simulink model "FW_Matlab_main"  (R2024b)
settings: Solver=ode4  StartTime=0.0  StopTime=inf  FixedStep=0.001  RelTol=1e-3
model workspace (MAT data in the model file):
  freq = 1
libraries: eeGeneralControl x8, slrealtimeiplib x5, cstblocks x3, simulink_extras x2, vrlib x1, aerolibanimutils x1, dspnetwork x1
(part 2 of 2)

== matlab function FW_Matlab_main/普通扑翼/MATLAB Function1 ==
  data: t input; y output
function y = back_flap(t)
%y=30+60*cos((226.08*t+180)*(pi/180));
y=60*cos((226.08*t+180)*(pi/180));
end

== matlab function FW_Matlab_main/普通扑翼/MATLAB Function2 ==
  data: t input; y output
function y = back_flap_twist(t)
  sita_u=90+30;   %上扑角度
  sita_d=90-30;   %下扑角度
  delta_T=0.4;
  T=1.6;
  sita_b_value=0;
  if t>=-delta_T/2 && t<=delta_T/2
    sita_b_value=(sita_u+sita_d)/2+((sita_u-sita_d)/2)*sin(3.14*t/delta_T);
  end
   if t>=delta_T/2 && t<=(T-delta_T)/2
    sita_b_value=sita_u;
   end
   if t>=(T-delta_T)/2 && t<=(T+delta_T)/2
    sita_b_value=(sita_u+sita_d)/2+((sita_u-sita_d)/2)*sin(3.14*(T/2-t)/delta_T);
   end
   if t>=(T+delta_T)/2 && t<=T-delta_T/2
    sita_b_value=sita_d;
   end
   if t>=T-delta_T/2 && t<=T
    sita_b_value=(sita_u+sita_d)/2+((sita_u-sita_d)/2)*sin(3.14*t/delta_T);
   end
   y=sita_b_value;
end

== matlab function FW_Matlab_main/普通扑翼/MATLAB Function3 ==
  data: t input; y output
function y = back_flap_twist(t)
  sita_u=90+30;   %上扑角度
  sita_d=90-30;   %下扑角度
  delta_T=0.4;
  T=1.6;
  sita_b_value=0;
  if t>=-delta_T/2 && t<=delta_T/2
    sita_b_value=(sita_u+sita_d)/2+((sita_u-sita_d)/2)*sin(3.14*t/delta_T);
  end
   if t>=delta_T/2 && t<=(T-delta_T)/2
    sita_b_value=sita_u;
   end
   if t>=(T-delta_T)/2 && t<=(T+delta_T)/2
    sita_b_value=(sita_u+sita_d)/2+((sita_u-sita_d)/2)*sin(3.14*(T/2-t)/delta_T);
   end
   if t>=(T+delta_T)/2 && t<=T-delta_T/2
    sita_b_value=sita_d;
   end
   if t>=T-delta_T/2 && t<=T
    sita_b_value=(sita_u+sita_d)/2+((sita_u-sita_d)/2)*sin(3.14*t/delta_T);
   end
   y=sita_b_value;
end

== matlab function FW_Matlab_main/Saw_Tooth ==
  data: freq input; Out output; t input
function Out = Saw_Tooth(freq,t)
% 设置参数
frequency = freq; % 频率
amplitude = 1 % 幅度

% 生成锯齿波形
Out = (sawtooth(2*pi*frequency*t, amplitude)+1)/2;

== matlab function FW_Matlab_main/蜻蜓扑动-VTOL模式 45度范围/MATLAB Function3 ==
  data: t input; y output
function y = back_flap_twist(t)
  sita_u=170;   %上扑角度
  sita_d=65;   %下扑角度
  delta_T=0.4;
  T=1.6;
  sita_b_value=0;
  if t>=-delta_T/2 && t<=delta_T/2
    sita_b_value=(sita_u+sita_d)/2+((sita_u-sita_d)/2)*sin(3.14*t/delta_T);
  end
   if t>=delta_T/2 && t<=(T-delta_T)/2
    sita_b_value=sita_u;
   end
   if t>=(T-delta_T)/2 && t<=(T+delta_T)/2
    sita_b_value=(sita_u+sita_d)/2+((sita_u-sita_d)/2)*sin(3.14*(T/2-t)/delta_T);
   end
   if t>=(T+delta_T)/2 && t<=T-delta_T/2
    sita_b_value=sita_d;
   end
   if t>=T-delta_T/2 && t<=T
    sita_b_value=(sita_u+sita_d)/2+((sita_u-sita_d)/2)*sin(3.14*t/delta_T);
   end
   y=sita_b_value;
end

== matlab function FW_Matlab_main/Saw_Tooth1 ==
  data: freq input; Out output; t input
function Out = Saw_Tooth(freq,t)
% 设置参数
frequency = freq; % 频率
amplitude = 1 % 幅度

% 生成锯齿波形
Out = (sawtooth(2*pi*frequency*t, amplitude)+1)/2;

== matlab function FW_Matlab_main/MATLAB Function ==
  data: Azimuth_Angle input; Freq_diff_out output; force_req_x input; force_req_y input
function Freq_diff_out = Flapping_Freq_Change(Azimuth_Angle,force_req_x,force_req_y)
%% 处理x轴
change_x=force_req_x/sind(Azimuth_Angle);
if isnan(change_x)
    change_x=0;
end
if isinf(change_x)
    change_x=0;
end

if abs(change_x)>10
  change_x=10;
end
Freq_diff_out_x=change_x;
%% 处理y轴
change_y=-force_req_y/cosd(Azimuth_Angle);
if isnan(change_y)
    change_y=0;
end
if isinf(change_y)
    change_y=0;
end

if abs(change_y)>10
  change_y=10;
end
Freq_diff_out_y=change_y;

Freq_diff_out=Freq_diff_out_x+Freq_diff_out_y;
if Freq_diff_out>=2.5
  Freq_diff_out=2.5;
end
if Freq_diff_out<=-2.5
  Freq_diff_out=-2.5;
end
end

== matlab function FW_Matlab_main/论文模式 FWR（拍幅：10//-10 扭转角5//25）Cl5.11? 升力没论文说的大 1/MATLAB Function ==
  data: t input; y output
function y = back_flap(t)
y=10*cos((226.08*t+180)*(pi/180));
end

== matlab function FW_Matlab_main/论文模式 FWR（拍幅：10//-10 扭转角5//25）Cl5.11? 升力没论文说的大 1/MATLAB Function1 ==
  data: t input; y output
function y = back_flap(t)
y=10*cos((226.08*t+180)*(pi/180));
end

== matlab function FW_Matlab_main/论文模式 FWR（拍幅：10//-10 扭转角5//25）Cl5.11? 升力没论文说的大 1/MATLAB Function2 ==
  data: t input; y output
function y = back_flap_twist(t)
  sita_u=90+25;   %上扑角度
  sita_d=90+5;   %下扑角度
  delta_T=0.4;
  T=1.6;
  sita_b_value=0;
  if t>=-delta_T/2 && t<=delta_T/2
    sita_b_value=(sita_u+sita_d)/2+((sita_u-sita_d)/2)*sin(3.14*t/delta_T);
  end
   if t>=delta_T/2 && t<=(T-delta_T)/2
    sita_b_value=sita_u;
   end
   if t>=(T-delta_T)/2 && t<=(T+delta_T)/2
    sita_b_value=(sita_u+sita_d)/2+((sita_u-sita_d)/2)*sin(3.14*(T/2-t)/delta_T);
   end
   if t>=(T+delta_T)/2 && t<=T-delta_T/2
    sita_b_value=sita_d;
   end
   if t>=T-delta_T/2 && t<=T
    sita_b_value=(sita_u+sita_d)/2+((sita_u-sita_d)/2)*sin(3.14*t/delta_T);
   end
   y=sita_b_value;
end

== matlab function FW_Matlab_main/论文模式 FWR（拍幅：10//-10 扭转角5//25）Cl5.11? 升力没论文说的大 1/MATLAB Function3 ==
  data: t input; y output
function y = back_flap_twist(t)
  sita_u=90+25;   %上扑角度
  sita_d=90+5;   %下扑角度
  delta_T=0.4;
  T=1.6;
  sita_b_value=0;
  if t>=-delta_T/2 && t<=delta_T/2
    sita_b_value=(sita_u+sita_d)/2+((sita_u-sita_d)/2)*sin(3.14*t/delta_T);
  end
   if t>=delta_T/2 && t<=(T-delta_T)/2
    sita_b_value=sita_u;
   end
   if t>=(T-delta_T)/2 && t<=(T+delta_T)/2
    sita_b_value=(sita_u+sita_d)/2+((sita_u-sita_d)/2)*sin(3.14*(T/2-t)/delta_T);
   end
   if t>=(T+delta_T)/2 && t<=T-delta_T/2
    sita_b_value=sita_d;
   end
   if t>=T-delta_T/2 && t<=T
    sita_b_value=(sita_u+sita_d)/2+((sita_u-sita_d)/2)*sin(3.14*t/delta_T);
   end
   y=sita_b_value;
end

== matlab function FW_Matlab_main/优化中 FWR（当前最优）10.29前/MATLAB Function ==
  data: t input; y output
function y = back_flap(t)
y=30+60*cos((226.08*t+180)*(pi/180));
end

== matlab function FW_Matlab_main/优化中 FWR（当前最优）10.29前/MATLAB Function1 ==
  data: t input; y output
function y = back_flap(t)
y=30+60*cos((226.08*t+180)*(pi/180));
end

== matlab function FW_Matlab_main/优化中 FWR（当前最优）10.29前/MATLAB Function2 ==
  data: t input; y output
function y = back_flap_twist(t)
  sita_u=90+45;   %上扑角度
  sita_d=90-5;   %下扑角度
  delta_T=0.4;
  T=1.6;
  sita_b_value=0;
  if t>=-delta_T/2 && t<=delta_T/2
    sita_b_value=(sita_u+sita_d)/2+((sita_u-sita_d)/2)*sin(3.14*t/delta_T);
  end
   if t>=delta_T/2 && t<=(T-delta_T)/2
    sita_b_value=sita_u;
   end
   if t>=(T-delta_T)/2 && t<=(T+delta_T)/2
    sita_b_value=(sita_u+sita_d)/2+((sita_u-sita_d)/2)*sin(3.14*(T/2-t)/delta_T);
   end
   if t>=(T+delta_T)/2 && t<=T-delta_T/2
    sita_b_value=sita_d;
   end
   if t>=T-delta_T/2 && t<=T
    sita_b_value=(sita_u+sita_d)/2+((sita_u-sita_d)/2)*sin(3.14*t/delta_T);
   end
   y=sita_b_value;
end

== matlab function FW_Matlab_main/蜻蜓扑动-FWR模式-角度与普通蜻蜓同  45度范围/MATLAB Function ==
  data: t input; y output
function y = back_flap(t)
y=15+30*cos((226.08*t+180)*(pi/180));
end

== matlab function FW_Matlab_main/优化中 FWR（当前最优）10.29前/MATLAB Function3 ==
  data: t input; y output
function y = back_flap_twist(t)
  sita_u=90+45;   %上扑角度
  sita_d=90-5;   %下扑角度
  delta_T=0.4;
  T=1.6;
  sita_b_value=0;
  if t>=-delta_T/2 && t<=delta_T/2
    sita_b_value=(sita_u+sita_d)/2+((sita_u-sita_d)/2)*sin(3.14*t/delta_T);
  end
   if t>=delta_T/2 && t<=(T-delta_T)/2
    sita_b_value=sita_u;
   end
   if t>=(T-delta_T)/2 && t<=(T+delta_T)/2
    sita_b_value=(sita_u+sita_d)/2+((sita_u-sita_d)/2)*sin(3.14*(T/2-t)/delta_T);
   end
   if t>=(T+delta_T)/2 && t<=T-delta_T/2
    sita_b_value=sita_d;
   end
   if t>=T-delta_T/2 && t<=T
    sita_b_value=(sita_u+sita_d)/2+((sita_u-sita_d)/2)*sin(3.14*t/delta_T);
   end
   y=sita_b_value;
end

== matlab function FW_Matlab_main/蜻蜓扑动-FWR模式-角度与普通蜻蜓同  45度范围/MATLAB Function1 ==
  data: t input; y output
function y = back_flap(t)
y=15+30*cos((226.08*t+180)*(pi/180));
end

== matlab function FW_Matlab_main/MATLAB Function6 ==
  data: Lift input; Cl output; freq input; Amp input
function Cl = Cl_cal(Lift,freq,Amp)
%初始参数设定
S=15*(1/100)*5.5*(1/100);
R2=0.5*18*(1/100);
Uref=2*deg2rad(Amp)*freq*R2;
air_p=1.225;
Cl=Lift*(1/1000)/(0.5*air_p*(Uref^2)*S);
end

== matlab function FW_Matlab_main/蜻蜓扑动-FWR模式-角度与普通蜻蜓同  45度范围/MATLAB Function2 ==
  data: t input; y output
function y = back_flap_twist(t)
  sita_u=170;   %上扑角度
  sita_d=65;   %下扑角度
  delta_T=0.4;
  T=1.6;
  sita_b_value=0;
  if t>=-delta_T/2 && t<=delta_T/2
    sita_b_value=(sita_u+sita_d)/2+((sita_u-sita_d)/2)*sin(3.14*t/delta_T);
  end
   if t>=delta_T/2 && t<=(T-delta_T)/2
    sita_b_value=sita_u;
   end
   if t>=(T-delta_T)/2 && t<=(T+delta_T)/2
    sita_b_value=(sita_u+sita_d)/2+((sita_u-sita_d)/2)*sin(3.14*(T/2-t)/delta_T);
   end
   if t>=(T+delta_T)/2 && t<=T-delta_T/2
    sita_b_value=sita_d;
   end
   if t>=T-delta_T/2 && t<=T
    sita_b_value=(sita_u+sita_d)/2+((sita_u-sita_d)/2)*sin(3.14*t/delta_T);
   end
   y=sita_b_value;
end

== matlab function FW_Matlab_main/蜻蜓扑动-FWR模式-角度与普通蜻蜓同  45度范围/MATLAB Function3 ==
  data: t input; y output
function y = back_flap_twist(t)
  sita_u=170;   %上扑角度
  sita_d=65;   %下扑角度
  delta_T=0.4;
  T=1.6;
  sita_b_value=0;
  if t>=-delta_T/2 && t<=delta_T/2
    sita_b_value=(sita_u+sita_d)/2+((sita_u-sita_d)/2)*sin(3.14*t/delta_T);
  end
   if t>=delta_T/2 && t<=(T-delta_T)/2
    sita_b_value=sita_u;
   end
   if t>=(T-delta_T)/2 && t<=(T+delta_T)/2
    sita_b_value=(sita_u+sita_d)/2+((sita_u-sita_d)/2)*sin(3.14*(T/2-t)/delta_T);
   end
   if t>=(T+delta_T)/2 && t<=T-delta_T/2
    sita_b_value=sita_d;
   end
   if t>=T-delta_T/2 && t<=T
    sita_b_value=(sita_u+sita_d)/2+((sita_u-sita_d)/2)*sin(3.14*t/delta_T);
   end
   y=sita_b_value;
end

== matlab function FW_Matlab_main/Msc 期间升力最大FWR模式 Msc 期间工作（拍幅：50//-20 扭转角10//50）/MATLAB Function ==
  data: t input; y output
function y = back_flap(t)
y=15+35*cos((226.08*t+180)*(pi/180));
end

== matlab function FW_Matlab_main/Msc 期间升力最大FWR模式 Msc 期间工作（拍幅：50//-20 扭转角10//50）/MATLAB Function1 ==
  data: t input; y output
function y = back_flap(t)
y=15+35*cos((226.08*t+180)*(pi/180));
end

== matlab function FW_Matlab_main/Msc 期间升力最大FWR模式 Msc 期间工作（拍幅：50//-20 扭转角10//50）/MATLAB Function2 ==
  data: t input; y output
function y = back_flap_twist(t)
  sita_u=90+50;   %上扑角度
  sita_d=90+10;   %下扑角度
  delta_T=0.4;
  T=1.6;
  sita_b_value=0;
  if t>=-delta_T/2 && t<=delta_T/2
    sita_b_value=(sita_u+sita_d)/2+((sita_u-sita_d)/2)*sin(3.14*t/delta_T);
  end
   if t>=delta_T/2 && t<=(T-delta_T)/2
    sita_b_value=sita_u;
   end
   if t>=(T-delta_T)/2 && t<=(T+delta_T)/2
    sita_b_value=(sita_u+sita_d)/2+((sita_u-sita_d)/2)*sin(3.14*(T/2-t)/delta_T);
   end
   if t>=(T+delta_T)/2 && t<=T-delta_T/2
    sita_b_value=sita_d;
   end
   if t>=T-delta_T/2 && t<=T
    sita_b_value=(sita_u+sita_d)/2+((sita_u-sita_d)/2)*sin(3.14*t/delta_T);
   end
   y=sita_b_value;
end

== matlab function FW_Matlab_main/Msc 期间升力最大FWR模式 Msc 期间工作（拍幅：50//-20 扭转角10//50）/MATLAB Function3 ==
  data: t input; y output
function y = back_flap_twist(t)
  sita_u=90+50;   %上扑角度
  sita_d=90+10;   %下扑角度
  delta_T=0.4;
  T=1.6;
  sita_b_value=0;
  if t>=-delta_T/2 && t<=delta_T/2
    sita_b_value=(sita_u+sita_d)/2+((sita_u-sita_d)/2)*sin(3.14*t/delta_T);
  end
   if t>=delta_T/2 && t<=(T-delta_T)/2
    sita_b_value=sita_u;
   end
   if t>=(T-delta_T)/2 && t<=(T+delta_T)/2
    sita_b_value=(sita_u+sita_d)/2+((sita_u-sita_d)/2)*sin(3.14*(T/2-t)/delta_T);
   end
   if t>=(T+delta_T)/2 && t<=T-delta_T/2
    sita_b_value=sita_d;
   end
   if t>=T-delta_T/2 && t<=T
    sita_b_value=(sita_u+sita_d)/2+((sita_u-sita_d)/2)*sin(3.14*t/delta_T);
   end
   y=sita_b_value;
end
